simulink model "ni_pci_test"  (Simulink 4.00)
settings: Solver=FixedStepDiscrete  SolverMode=SingleTasking  StartTime=0.0  StopTime=10.0  RelTol=1e-3
libraries: ni_pci x11
settings Model: Creator=root  LastModifiedBy=root  SaveTime=off  SaveOutput=off  MaxDataPoints=20000  SimulationMode=external  RTWSystemTargetFile=grt_rtai.tlc  RTWOptions="-aBasePriority=30 -aExtMode=1 -aForceParamTrailComments=0 -aInlineInvariantSignals=0 -aInlineParameters=0 -aLocalBlockOutputs=1 -aLogVarNameModifier=\"rt_\" -aMatFileLogging=0 -aRTWVerbose=1 -aRollThreshold=5 -aShowEliminatedStatements=1 -aTaskStackSize=16384"  RTWTemplateMakefile=grt_rtai.tmf  ExtModeTrigDuration=10000  BlockReductionOpt=off

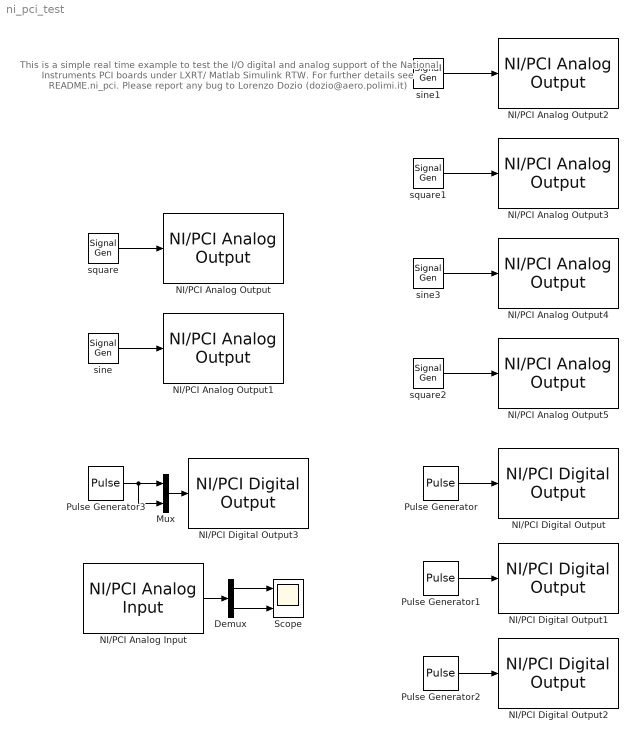
== system ni_pci_test ==
  note: This is a simple real time example to test the
      | I/O digital and analog support
      | of the National Instruments PCI boards
      | under LXRT/ Matlab Simulink RTW.
      | For further details see README.ni_pci.
      |
      | Please report any bug to Lorenzo Dozio
      | (dozio@aero.polimi.it)
  Demux : Demux  Outputs=2  BusSelectionMode=off
  Mux : Mux  Inputs=2
  NI/PCI Analog Input : ni_pci/NI//PCI Analog Input  index=0  nchan=2  chantype=RSE  gain=0.5  pol=bipolar  dither=off  dt=0.0001
  NI/PCI Analog Output : ni_pci/NI//PCI Analog Output  index=0  dacsel=DAC0  dacref=internal  dacpol=bipolar  dt=0.0001
  NI/PCI Analog Output1 : ni_pci/NI//PCI Analog Output  index=0  dacsel=DAC1  dacref=internal  dacpol=bipolar  dt=0.0001
  NI/PCI Analog Output2 : ni_pci/NI//PCI Analog Output  index=1  dacsel=DAC1  dacref=internal  dacpol=bipolar  dt=0.0001
  NI/PCI Analog Output3 : ni_pci/NI//PCI Analog Output  index=1  dacsel=DAC2  dacref=internal  dacpol=bipolar  dt=0.0001
  NI/PCI Analog Output4 : ni_pci/NI//PCI Analog Output  index=1  dacsel=DAC3  dacref=internal  dacpol=bipolar  dt=0.0001
  NI/PCI Analog Output5 : ni_pci/NI//PCI Analog Output  index=1  dacsel=DAC4  dacref=internal  dacpol=bipolar  dt=0.0001
  NI/PCI Digital Output : ni_pci/NI//PCI Digital Output  index=1  dio_82C55=off  port=C_low  nchan=1  dio_module=on  line=0  dt=0.0001
  NI/PCI Digital Output1 : ni_pci/NI//PCI Digital Output  index=1  dio_82C55=off  port=C_low  nchan=1  dio_module=on  line=1  dt=0.0001
  NI/PCI Digital Output2 : ni_pci/NI//PCI Digital Output  index=1  dio_82C55=off  port=C_low  nchan=1  dio_module=on  line=2  dt=0.0001
  NI/PCI Digital Output3 : ni_pci/NI//PCI Digital Output  index=0  dio_82C55=on  port=B  nchan=2  dio_module=off  line=0  dt=0.0001
  Pulse Generator : DiscretePulseGenerator  Amplitude=0.5  Period=50  PulseWidth=10  PhaseDelay=0  SampleTime=0.0001
  Pulse Generator1 : DiscretePulseGenerator  Amplitude=0.5  Period=50  PulseWidth=40  PhaseDelay=0  SampleTime=0.0001
  Pulse Generator2 : DiscretePulseGenerator  Amplitude=0.5  Period=50  PulseWidth=25  PhaseDelay=0  SampleTime=0.0001
  Pulse Generator3 : DiscretePulseGenerator  Amplitude=0.5  Period=50  PulseWidth=10  PhaseDelay=0  SampleTime=0.0001
  Scope : Scope  NumInputPorts=2
      settings: TimeRange=0.1  YMin=-10~-10  YMax=10~10  SaveToWorkspace=off  SaveName=ScopeData  MaxDataPoints=5000
  sine : SignalGenerator  WaveForm=sine  Amplitude=5  Frequency=50  Units=Hertz
  sine1 : SignalGenerator  WaveForm=sine  Amplitude=5  Frequency=50  Units=Hertz
  sine3 : SignalGenerator  WaveForm=sine  Amplitude=5  Frequency=10  Units=Hertz
  square : SignalGenerator  WaveForm=square  Amplitude=2  Frequency=30  Units=Hertz
  square1 : SignalGenerator  WaveForm=square  Amplitude=2  Frequency=30  Units=Hertz
  square2 : SignalGenerator  WaveForm=square  Amplitude=2  Frequency=100  Units=Hertz
  wires:
  square/1 -> NI/PCI Analog Output/1
  sine1/1 -> NI/PCI Analog Output2/1
  square1/1 -> NI/PCI Analog Output3/1
  sine3/1 -> NI/PCI Analog Output4/1
  sine/1 -> NI/PCI Analog Output1/1
  square2/1 -> NI/PCI Analog Output5/1
  Pulse Generator/1 -> NI/PCI Digital Output/1
  Pulse Generator1/1 -> NI/PCI Digital Output1/1
  Pulse Generator2/1 -> NI/PCI Digital Output2/1
  Pulse Generator3/1 -> Mux/1, Mux/2
  Mux/1 -> NI/PCI Digital Output3/1
  NI/PCI Analog Input/1 -> Demux/1
  Demux/1 -> Scope/1
  Demux/2 -> Scope/2
